simulink model "f_updated_vehicle_model"  (R2025b)
settings: Solver=ode23tb  StartTime=0.0  StopTime=20  MaxStep=0.001  RelTol=1e-3
model workspace (MAT data in the model file):
  init_r = 0
  init_vx = 0
  init_vy = 0
values from neighbouring files (symbols this model uses):
  Par =     [0_Load_data.mat]
  TireData =     [0_Load_data.mat]
undefined symbols (not defined in the file or in its folder): aero_par, Battery, Motor, SimInput_Steer, SimInput_TorqueFL, SimInput_TorqueFR, SimInput_TorqueRL, SimInput_TorqueRR, sus_par
libraries: simulink x3, BatteryEstimators x1
(part 2 of 2)

== matlab function f_updated_vehicle_model/roll and pitch angles/Phi_constants ==
  data: K_phi output; C_phi output; sus_par parameter; Par parameter
function [K_phi,C_phi] = fcn(sus_par,Par)

% Calculating Pitching stiffness
Kw_fl = sus_par.Ks_f.*(sus_par.Motion_ratio_f)^2; 
Kw_fr = sus_par.Ks_f.*(sus_par.Motion_ratio_f)^2;
Kw_rl = sus_par.Ks_r.*(sus_par.Motion_ratio_r)^2;
Kw_rr = sus_par.Ks_r.*(sus_par.Motion_ratio_r)^2;

K_phi = (Kw_fl + Kw_fr).*(Par.Tf/2)^2 + (Kw_rl + Kw_rr).*(Par.Tr/2)^2;

% Calculating Pitch Damping
Cw_fl = sus_par.C_damp_f.*(sus_par.Motion_ratio_f)^2;
Cw_fr = sus_par.C_damp_f.*(sus_par.Motion_ratio_f)^2;
Cw_rl = sus_par.C_damp_r.*(sus_par.Motion_ratio_r)^2;
Cw_rr = sus_par.C_damp_r.*(sus_par.Motion_ratio_r)^2;

C_phi = (Cw_fl + Cw_fr).*(Par.Tf/2)^2 + (Cw_rl + Cw_rr).*(Par.Tr/2)^2;

== matlab function f_updated_vehicle_model/Battery Pack/MATLAB Function ==
  data: Voc_pack input; v_bus output; R0_pack input; V_rc input; I_dc input
function v_bus = fcn(Voc_pack, R0_pack, V_rc, I_dc)
    % This function calculates the terminal voltage of the battery pack.
    % Voc_pack: Output from OCV LUT multiplied by Ns
    % R0_pack:  Output from R0 LUT multiplied by (Ns/Np)
    % V_rc:     Instantaneous voltage across the RC branch
    % I_dc:     Total DC current from the motor

    % 1. Calculate the instantaneous Ohmic drop (Ohm's Law)
    V_ohmic = I_dc * R0_pack;

    % 2. Calculate terminal voltage (Vt = Voc - V_ohmic - V_rc)
    v_bus = Voc_pack - V_ohmic - V_rc;

    % 3. Safety: Ensure voltage doesn't drop below a physical floor (e.g., 2.5V * Ns)
    % This prevents simulation crashes if the battery is fully depleted.
    v_bus = max(v_bus, 2.5 * 144); 
end

== matlab function f_updated_vehicle_model/Brakes/MATLAB Function ==
  data: brake_pedal input; T_brakes output; omega input; Brake parameter
function T_brakes = fcn(brake_pedal, omega, Brake)
    % BRAKE TORQUE CALCULATION
    % Converts normalized pedal/actuator position into physical torque
    % and ensures torque direction opposes wheel rotation.
    
    % 1. Calculate Magnitude of Torque based on Command (0-1)
    % We use the static max targets from the design sheet
    T_mag_Front = brake_pedal * Brake.MaxTorque_Wheel_F;
    T_mag_Rear  = brake_pedal * Brake.MaxTorque_Wheel_R;
    
    % Initialize output vector (FL, FR, RL, RR)
    T_brakes = zeros(1, 4);
    
    % 2. Apply Torque per Wheel with Directional Logic
    % Loop through all 4 wheels to apply logic individually
    % Indices: 1=FL, 2=FR, 3=RL, 4=RR
    
    for i = 1:4
        % Determine if this is a Front (1,2) or Rear (3,4) wheel
        if i <= 2
            T_req = T_mag_Front;
        else
            T_req = T_mag_Rear;
        end
        
        % Directional Check:
        % Torque must be negative if omega is positive, and vice versa.
        % -sign(omega) flips the torque direction.
        T_applied = T_req * -sign(omega(i));
        
        % Zero-Speed Cutoff:
        % If wheel is nearly stopped, clamp torque to zero to prevent 
        % the simulation from "driving" the car backwards.
        if abs(omega(i)) < Brake.ZeroSpeedThreshold
            T_applied = 0;
            
            % Advanced: Ideally, below threshold, T_brake should act as 
            % a viscous damper or Coulomb friction that exactly cancels 
            % remaining motion, but zeroing is sufficient for laptime sims.
        end
        
        T_brakes(i) = T_applied;
    end
end

== matlab function f_updated_vehicle_model/Motor/MATLAB Function ==
  data: rpm input; Torque_Nm output; throttle input; v_dc input
function Torque_Nm = fcn(rpm, throttle, v_dc)
    % 1. Constants
    p = 4;                      % Pole pairs 
    L = 0.393e-3;               % Inductance
    kt = 0.492;
    psi_m = kt/(1.5*p*sqrt(2));              % Flux linkage derived from kt
    I_lim = 61; % Peak phase current 
    V_max = v_dc / sqrt(3);     % Maximum available phase voltage
    
    % 2. Speed Conversion
    omega_m = rpm * (2*pi/60);
    omega_e = p * omega_m;
    
    % 3. MTPA / Field Weakening Logic
    if omega_e < 1e-3 % Handle standstill
        iq = I_lim* sqrt(2) * throttle;
        id = 0;
    else
        % Calculate required voltage for MTPA (id=0)
        V_req = omega_e * sqrt((L*I_lim)^2 + psi_m^2);
        
        if V_req <= V_max
            % Below base speed
            iq = I_lim;
            id = 0;
        else
            % Above base speed (Field Weakening)
            % Solving the quadratic for iq at the boundary of V_max and I_lim
            a = (omega_e * L)^2;
            b = 2 * omega_e^2 * L * psi_m;
            c = (omega_e * psi_m)^2 + (omega_e * L * I_lim)^2 - V_max^2;
            
            % Simple analytical approximation for constant power region
            iq = min(I_lim, V_max / (omega_e * L));
        end
    end
    
    % 4. Final Torque Calculation (with 29.1 Nm cap)
    Torque_Nm = min(29.1, 1.5 * p * psi_m * iq / sqrt(2)); 
end

== matlab function f_updated_vehicle_model/Normal Loads ==
  data: Fz_out output; phi input; theta input; Kw input; Vel input; Par parameter; Fs output size=4; Farb output; F_aero_total output; Zs output; aero_par parameter; sus_par parameter
function [Fz_out,Fs,Farb,F_aero_total,Zs] = fcn(phi,theta,Kw,Vel,Par,aero_par,sus_par)
    %#codegen
    % Inputs:
    %   ax_g, ay_g : Acceleration 
    %   m          : Mass [kg]
    %   Par        : Structure with field .g, .WB, .TW, .CG_h, .WD_R, .K_roll_F

    % 1. Constants
    g = Par.g;
    L = Par.WB;    % Wheelbase
    Tf = Par.Tf;   % Front track width
    Tr = Par.Tr;   % Rear Track width
    h = Par.CG_h;  % CG Height
    m = Par.m;
   
    % Front and rear Wheelbase
    Lf = L*0.51;  % Front wheel base
    Lr = L*0.49;  % Rear wheel base

    % Static load 
    F_static = m*g;  

    % Stiffness at each wheel:
    Kt = 90000;
    stiff_1 = Kw(1)*Kt/(Kw(1)+Kt);
    stiff_2 = Kw(2)*Kt/(Kw(2)+Kt);
    stiff_3 = Kw(3)*Kt/(Kw(3)+Kt);
    stiff_4 = Kw(4)*Kt/(Kw(4)+Kt);

    % F_aero = 0.5 * rho * Cl * A * v^2
    F_aero_total = -0.5 * aero_par.rho * aero_par.Cl * aero_par.Area * Vel^2;
    
    % Vertical deflection of each suspension(compression = -ve)
    zsfl = Lf*theta + (Tf/2)*phi - 0.5 * F_aero_total * (1 - aero_par.CP_rear)/stiff_1;
    zsfr = Lf*theta - (Tf/2)*phi - 0.5 * F_aero_total * (1 - aero_par.CP_rear)/stiff_2;
    zsrl = -Lr*theta + (Tr/2)*phi - 0.5 * F_aero_total*(aero_par.CP_rear)/stiff_3;
    zsrr = -Lr*theta - (Tr/2)*phi - 0.5 * F_aero_total*(aero_par.CP_rear)/stiff_4;

    Zs = [zsfl;zsfr;zsrl;zsrr];

    % Spring force at each wheel
    Fs_fl = stiff_1*zsfl;
    Fs_fr = stiff_2*zsfr;
    Fs_rl = stiff_3*zsrl;
    Fs_rr = stiff_4*zsrr;

    % Calculation of Anti roll bar forces at each wheel
    delta_zf = zsfl - zsfr;
    delta_zr = zsrl - zsrr;

    F_arb_fl = sus_par.K_arb_f*delta_zf/2;
    F_arb_fr = -sus_par.K_arb_f*delta_zf/2;
    F_arb_rl = sus_par.K_arb_r*delta_zr/2;
    F_arb_rr = -sus_par.K_arb_r*delta_zr/2;

    % Net normal force on each wheel
    F_static_per_wheel = F_static/4;

    Fz_FL = F_static_per_wheel - Fs_fl - F_arb_fl;
    Fz_FR = F_static_per_wheel - Fs_fr - F_arb_fr;
    Fz_RL = F_static_per_wheel - Fs_rl - F_arb_rl;
    Fz_RR = F_static_per_wheel - Fs_rr - F_arb_rr;
   
    % Safety Clamp (Wheelie prevention)
    Min_Load = 10; 

    Fz_FL = max(Fz_FL, Min_Load);
    Fz_FR = max(Fz_FR, Min_Load);
    Fz_RL = max(Fz_RL, Min_Load);
    Fz_RR = max(Fz_RR, Min_Load);

    Fz_out = [Fz_FL; Fz_FR; Fz_RL; Fz_RR];
    
    Fs = [Fs_fl;Fs_fr;Fs_rl;Fs_rr];
    Farb = [F_arb_fl;F_arb_fr;F_arb_rl;F_arb_rr];

% Distribute Aero (Usually based on Center of Pressure, CP)
   % 
   % aero_Fz_FL = Fz_FL + ;
   % aero_Fz_FR = Fz_FR + ;
   % aero_Fz_RL = Fz_RL + ;
   % aero_Fz_RR = Fz_RR + ;

   % Fz_new = [aero_Fz_FL;aero_Fz_FR;aero_Fz_RL;aero_Fz_RR];
   
   
end

== matlab function f_updated_vehicle_model/Motor/MATLAB Function1 ==
  data: rpm_feedback input; Torque_Nm output; throttle input; v_dc_bus input
function Torque_Nm = fcn(rpm_feedback, throttle, v_dc_bus)
    % --- 1. Define Motor Constants from Datasheet ---
    p = 4;                          % Number of pole pairs 
    L = 0.393e-3;                   % Phase inductance in Henries 
    kt = 0.492;                     % Torque constant in Nm/Arms 
    psi_m = kt / (1.5 * p * sqrt(2)); % Calculate magnet flux linkage (~0.058 Wb)
    I_max_rms = 61;                 % Maximum peak current in Arms 
    n_max = 20000;                  % Maximum mechanical RPM limit 
    T_peak_limit = 29.1;            % Absolute peak torque cap in Nm 

    % --- 2. Enforce Hard Mechanical RPM Limit ---
    if abs(rpm_feedback) >= n_max   % Check if current speed exceeds mechanical redline
        Torque_Nm = 0;              % Kill all torque production at the limit
        return;                     % Exit function immediately
    end

    % --- 3. Convert Inputs to Electrical Units ---
    omega_m = rpm_feedback * (2*pi/60);      % Convert mechanical RPM to rad/s
    omega_e = omega_m * p;                   % Convert mechanical speed to electrical frequency
    V_max_phase = v_dc_bus / sqrt(3);        % Calculate max phase voltage (fundamental limit)
    I_cmd_peak = I_max_rms * sqrt(2) * throttle; % Scaled peak current command based on throttle

    % --- 4. Determine Operating Region (MTPA vs. Field Weakening) ---
    % Calculate the voltage required for MTPA (where id = 0)
    % Equation: V = omega_e * sqrt( (L*iq)^2 + (psi_m)^2 )
    V_required_mtpa = abs(omega_e) * sqrt((L * I_cmd_peak)^2 + psi_m^2);

    if V_required_mtpa <= V_max_phase        % If enough voltage is available for requested torque
        % REGION 1: Below Base Speed (Maximum Torque Per Ampere)
        id = 0;                              % No d-axis current needed (standard operation)
        iq = I_cmd_peak;                     % All available current used for torque production
    else
        % REGION 2: Above Base Speed (Field Weakening)
        % We must inject negative d-axis current (id) to oppose psi_m and stay within V_max
        % Intersection of Current Circle (id^2 + iq^2 = I^2) and Voltage Ellipse
        
        % Solving the voltage ellipse for id:
        % (V_max/omega_e)^2 = (L*iq)^2 + (L*id + psi_m)^2
        % This simplifies to a quadratic equation for id
        a_quad = L^2;                        % Quadratic coefficient 'a'
        b_quad = 2 * L * psi_m;              % Quadratic coefficient 'b'
        c_quad = psi_m^2 + (L * I_cmd_peak)^2 - (V_max_phase / omega_e)^2; % Coefficient 'c'
        
        % Calculate the required negative d-axis current using the quadratic formula
        id = (-b_quad + sqrt(b_quad^2 - 4 * a_quad * c_quad)) / (2 * a_quad);
        
        % Enforce physical bounds on current components
        id = max(min(id, 0), -I_cmd_peak);   % Clamp id between -I_max and 0
        iq = sqrt(max(0, I_cmd_peak^2 - id^2)); % Solve for remaining q-axis current
    end

    % --- 5. Calculate Final Torque Output ---
    % Standard PMSM Torque Equation: Te = 1.5 * p * psi_m * iq
    T_generated = 1.5 * p * psi_m * iq;      % Calculate the raw electromagnetic torque
    
    % Final output is capped by the mechanical peak torque of the motor
    Torque_Nm = min(T_generated, T_peak_limit); % Saturate at 29.1 Nm 
end

== matlab function f_updated_vehicle_model/Motor/Motor with Field Weakening ==
  data: rpm_feedback input; Torque_Nm output; throttle input; v_dc_bus input; Motor parameter; I_dc output
function [Torque_Nm, I_dc] = fcn(rpm_feedback, throttle, v_dc_bus, Motor)
    % HIGH-FIDELITY PMSM MOTOR MODEL
    % Inputs:
    %   rpm_feedback : Instantaneous wheel speed * gear ratio [rpm]
    %   throttle     : Driver input signal [0 to 1]
    %   v_dc_bus     : Instantaneous voltage from battery pack [V]
    %   Motor        : Struct containing constants (kt, L, p, n_max, etc.)
    
    % --- 1. Enforce Mechanical Redline ---
    % n_max is 20,000 rpm per datasheet.
    if abs(rpm_feedback) >= Motor.n_max
        Torque_Nm = 0;
        I_dc = 0;
        return;
    end

    % --- 2. Electrical Conversions ---
    omega_m = rpm_feedback * (2*pi/60);          % Mechanical rad/s
    omega_e = abs(omega_m * Motor.p);            % Electrical frequency 
    V_max_phase = v_dc_bus / sqrt(3);            % Max phase voltage (fundamental limit)
    I_cmd_peak = Motor.I_max_rms * sqrt(2) * throttle; % Commanded peak current 

    % --- 3. Region Selection: MTPA vs Field Weakening ---
    % Calculate voltage required for id=0 operation (Maximum Torque Per Ampere)
    % psi_m is the flux linkage derived from kt (~0.492 Nm/A).
    V_req_mtpa = omega_e * sqrt((Motor.L * I_cmd_peak)^2 + Motor.psi_m^2);

    if V_req_mtpa <= V_max_phase
        % REGION 1: Below Base Speed
        id = 0;
        iq = I_cmd_peak;
    else
        % REGION 2: Above Base Speed (Field Weakening)
        % Intersecting the Current Circle (id^2 + iq^2 = Imax^2) with the Voltage Ellipse.
        % Solving the quadratic for d-axis current (id).
        a = Motor.L^2;
        b = 2 * Motor.L * Motor.psi_m;
        c = Motor.psi_m^2 + (Motor.L * I_cmd_peak)^2 - (V_max_phase / max(omega_e(3), 0.1))^2;
        
        % Solve for negative id to oppose magnet flux
        id = (-b + sqrt(b^2 - 4 * a * c)) / (2 * a);
        
        % Ensure id is within physical bounds and calculate remaining iq
        id = max(min(id, 0), -I_cmd_peak); 
        iq = sqrt(max(0, I_cmd_peak^2 - id^2));
    end

    % --- 4. Torque Calculation ---
    % Te = 1.5 * p * psi_m * iq
    T_generated = 1.5 * Motor.p * Motor.psi_m * iq;
    
    % Cap at peak mechanical torque (29.1 Nm)[cite: 8, 136].
    Torque_Nm = min(T_generated, Motor.T_peak_limit);

    % --- 5. DC Current Calculation (The Battery Interaction) ---
    % Mechanical Output Power
    P_mech = abs(Torque_Nm * omega_m(3));
    
    % Copper Losses (3 * R_phase * I_rms^2) 
    % R_phase = 0.126 Ohm per datasheet.
    P_copper = 3 * 0.126 * (I_cmd_peak / sqrt(2))^2;
    
    % Total electrical power requested from the battery
    P_elec_total = P_mech + P_copper;
    
    % Calculate DC current draw (I = P/V)
    if v_dc_bus > 10
        I_dc = P_elec_total / v_dc_bus;
    else
        I_dc = 0;
    end
end

== matlab function f_updated_vehicle_model/Torque Distribution/MATLAB Function ==
  data: T_wheel input; T_FL output; T_brake_vec input; T_FR output; T_RL output; T_RR output
function [T_FL, T_FR, T_RL, T_RR] = torque_combiner(T_wheel, T_brake_vec)
    % T_brake_vec is a 4x1 input: [FL; FR; RL; RR]
    
    % Front Wheels: Brake only
    T_FL = -T_brake_vec(1);
    T_FR = -T_brake_vec(2);
    
    % Rear Wheels: (Motor / 2) - Brake
    % Assuming 50/50 torque split from an open diff
    T_RL = (T_wheel) - T_brake_vec(3);
    T_RR = (T_wheel) - T_brake_vec(4);
end

== matlab function f_updated_vehicle_model/Simplified Tire Model ==
  data: Fz input; Fx output size=4; slip_ratios input; slip_angles input; camber_angles input; Fy output size=4; Mz output size=4; Mu_x output size=4; Mu_y output size=4; TireData parameter; Par parameter; sus_par parameter
function [Fx, Fy, Mz, Mu_x, Mu_y] = fcn(Fz, slip_ratios, slip_angles, camber_angles, TireData,Par,sus_par)
%#codegen
% =========================================================================
%  VECTORIZED MAGIC FORMULA 5.2 (4-WHEEL)
%  Computes tire physics for all 4 corners simultaneously using element-wise math.
%
%  INPUTS (All 4x1 Vectors):
%    Fz    : Vertical Loads [N] -> [FL; FR; RL; RR]
%    Kappa : Slip Ratios [-]
%    Alpha : Slip Angles [rad]
%    Gamma : Camber Angles [rad]
%    TireData : Parameter Struct (Must be loaded in Base Workspace)
%
%  OUTPUTS (All 4x1 Vectors):
%    Fx    : Longitudinal Force [N]
%    Fy    : Lateral Force [N]
%    Mz    : Self-Aligning Torque [Nm]
%    Mu_x  : Long. Friction Coeff [-]
%    Mu_y  : Lat. Friction Coeff [-]
% =========================================================================

    % 1. EXTRACT PARAMETERS (Scalars)
    p = TireData;
    s = TireData.Scales;
    Fz0 = Par.Fz0;
    Rw  = Par.R0;
    
    % 2. INPUT SAFETY & NORMALIZATION
    % Clamp negative loads to 0 (Tires can't pull ground)
    Fz_safe = max(Fz, 0); 
    
    % Avoid division by zero for Mu calculations later
    Fz_denom = max(Fz_safe, 1.0); 

    % Normalized Load (dfz) - Vectorized
    dfz = (Fz_safe - Fz0) ./ Fz0;

    % ---------------------------------------------------------------------
    % A. LONGITUDINAL FORCE (Fx) - VECTORIZED
    % ---------------------------------------------------------------------
    Cx = p.PCX1 * s.LCX;
    
    % Friction Coeff Mu_x
    mu_x_base = (p.PDX1 + p.PDX2 .* dfz) .* (1 - p.PDX3 .* camber_angles.^2) .* s.LMUX;
    Dx = mu_x_base .* Fz_safe;
    
    % Stiffness Kx
    Kx = Fz_safe .* (p.PKX1 + p.PKX2 .* dfz) .* exp(p.PKX3 .* dfz) .* s.LKX;
    
    % Stiffness Factor Bx
    Bx = Kx ./ (Cx .* Dx + 1e-6); 
    
    % Shifts (Horizontal & Vertical)
    Shx = (p.PHX1 + p.PHX2 .* dfz) .* s.LHX;
    Svx = Fz_safe .* (p.PVX1 + p.PVX2 .* dfz) .* s.LVX;
    
    % Composite Slip
    k_s = slip_ratios + Shx;
    
    % Curvature Ex (Sign Dependent)
    Ex = (p.PEX1 + p.PEX2 .* dfz + p.PEX3 .* dfz.^2) .* (1 - p.PEX4 .* sign(k_s)) .* s.LEX;
    Ex(Ex > 1) = 1; % Clamp
    
    % Calculation
    Bx_k = Bx .* k_s;
    Fx = Dx .* sin(Cx .* atan(Bx_k - Ex .* (Bx_k - atan(Bx_k)))) + Svx;

    % ---------------------------------------------------------------------
    % B. LATERAL FORCE (Fy) - VECTORIZED
    % ---------------------------------------------------------------------
    Cy = p.PCY1 * s.LCY;
    
    % Friction Coeff Mu_y
    mu_y_base = (p.PDY1 + p.PDY2 .* dfz) .* (1 - p.PDY3 .* camber_angles.^2) .* s.LMUY;
    Dy = mu_y_base .* Fz_safe;
    
    % Cornering Stiffness Ky (Trig Form)
    Ky = p.PKY1 .* Fz0 .* sin(2 .* atan(Fz_safe ./ (p.PKY2 .* Fz0))) .* (1 - p.PKY3 .* abs(camber_angles)) .* s.LKY;
    
    % Poly fallback check (if PKY2 implies poly form)
    if (Ky(1) < 1)
        Ky = Fz_safe .* (p.PKY1 + p.PKY2 .* dfz) .* s.LKY;
    end
    
    By = Ky ./ (Cy .* Dy + 1e-6);
    
    % Shifts
    Shy = (p.PHY1 + p.PHY2 .* dfz) .* s.LHY;
    Svy = Fz_safe .* (p.PVY1 + p.PVY2 .* dfz) .* s.LVY;
    
    a_s = slip_angles + 0*Shy;
    
    % Curvature Ey (Sign Dependent)
    Ey = (p.PEY1 + p.PEY2 .* dfz) .* (1 - (p.PEY3 + p.PEY4 .* camber_angles) .* sign(a_s)) .* s.LEY;
    Ey(Ey > 1) = 1;
    
    % Calculation
    By_a = By .* a_s;
    Fy = -(Dy .* sin(Cy .* atan(By_a - Ey .* (By_a - atan(By_a)))) + 0*Svy);

    % ---------------------------------------------------------------------
    % C. SELF-ALIGNING TORQUE (Mz) - VECTORIZED
    % ---------------------------------------------------------------------
    % Peak Trail Dt
    Dt = (p.QDZ1 + p.QDZ2 .* dfz) .* (1 - p.QDZ3 .* abs(camber_angles)) .* Rw .* s.LTR;
    
    % Trail Slope Bt
    Bt = (p.QBZ1 + p.QBZ2 .* dfz + p.QBZ3 .* dfz.^2) .* (1 + p.QBZ4 .* abs(camber_angles)) .* (s.LKY / s.LMUY);
    
    Ct = p.QCZ1; % Scalar
    Et = (p.QEZ1 + p.QEZ2 .* dfz + p.QEZ3 .* dfz.^2);
    
    % Trail 't' Calculation(Pneumatic trail)
    Bt_a = Bt .* a_s;
    alpha_t = Bt_a - Et .* (Bt_a - atan(Bt_a));
    t = Dt .* cos(Ct .* atan(alpha_t)) .* cos(a_s);

    % Trail 'tm' Calculation(mechanical trail)
    tm = Rw.*tan(sus_par.Caster_static);

    % Residual Mzr
    Dr = Fz_safe .* Rw .* (p.QDZ6 + p.QDZ7 .* dfz) .* s.LRES;
    Br = 10;
    Mzr = Dr .* cos(atan(Br .* a_s));
    
    % Final Mz (Standard Restoring: Negative Slope)
    % Note: If you want positive slope (sharp tune from before), multiply term by -1.
    Mz = -(t+tm).*Fy + Mzr;

    % ---------------------------------------------------------------------
    % D. OUTPUTS (Zero out lifted wheels)
    % ---------------------------------------------------------------------
    % Friction Coeffs
    Mu_x = Fx ./ Fz_denom;
    Mu_y = Fy ./ Fz_denom;

    % Clean up lifted wheels (Fz <= 0)
    % lifted_idx = Fz <= 0;
    % Fx(lifted_idx) = 0;
    % Fy(lifted_idx) = 0;
    % Mz(lifted_idx) = 0;
    % Mu_x(lifted_idx) = 0;
    % Mu_y(lifted_idx) = 0;

end

== matlab function f_updated_vehicle_model/slip ratios ==
  data: Vx input; Vy input; slip_ratios output; yawrate input; Omega input; Steer_FL input; Steer_FR input; Par parameter
function slip_ratios = fcn(Vx,Vy, yawrate, Omega,Steer_FL,Steer_FR, Par)
%#codegen


    % 1. Constants
    Tf = Par.Tf;
    Tr = Par.Tr;
    Rw = Par.R0;
    
    a = Par.Lf;
    b = Par.Lr;
    r = yawrate;
    % 2 Yaw Rate Correction (Kinematics)
    
    Vx_FL = Vx - yawrate * (Tf/2);  % Front Left
    Vx_FR = Vx + yawrate * (Tf/2);  % Fron Right
    Vx_RL = Vx - yawrate * (Tr/2);  % Rear Left
    Vx_RR = Vx + yawrate * (Tr/2);  % Rear Right
    
    Vx_vec = [Vx_FL; Vx_FR; Vx_RL; Vx_RR];
    
    Vy_FL = Vy + r * a;
    Vy_FR = Vy+ r * a;
    Vy_RL = Vy- r * b;
    Vy_RR = Vy- r * b;

    Vy_vec = [Vy_FL; Vy_FR; Vy_RL; Vy_RR];
    Delta = [Steer_FL;Steer_FR;0;0];
    % 3. Slip Angle Correction (Projection)
 
    V_road_plane = Vx_vec .* cos(Delta) + Vy_vec .* sin(Delta);

    % 4. Calculate Wheel Linear Speed
    V_wheel = Omega .* Rw;

    % 5. Calculate Slip Ratio
    V_safe_threshold = 0.1; 
    V_ref = max(abs(V_road_plane), V_safe_threshold);
    
    slip_ratios_raw = (V_wheel - V_road_plane) ./ V_ref;
    slip_ratios = min(max(slip_ratios_raw,-1),1);
end

== matlab function f_updated_vehicle_model/Slip Angles ==
  data: Vx input; slip_angles output; Vy input; yawrate input; Steer_FL input; Steer_FR input; Par parameter
function slip_angles = fcn(Vx, Vy, yawrate, Steer_FL, Steer_FR, Par)
%#codegen

    % 1. Geometry Setup
    T = Par.Tf;
    
    % Distance from CG to Axles
    a = Par.Lf;     
    b = Par.Lr;             
    half_T = T / 2;

    % 2. Calculate Velocity Components at Each Corner
    % Kinematic transformation from CG to Hubs
    % Front Left (1)
        Vx_FL = Vx - yawrate * half_T;
        Vy_FL = Vy + yawrate * a;
    
    % Front Right (2)
        Vx_FR = Vx + yawrate * half_T;
        Vy_FR = Vy + yawrate * a;
    
    % Rear Left (3)
        Vx_RL = Vx - yawrate * half_T;
        Vy_RL = Vy - yawrate * b;
    
    % Rear Right (4)
        Vx_RR = Vx + yawrate * half_T;
        Vy_RR = Vy - yawrate * b;

    % 3. Calculate Velocity Angles (Theta_V)

        Theta_FL = atan2(Vy_FL, max(Vx_FL,0.1)); 
        Theta_FR = atan2(Vy_FR, max(Vx_FR,0.1));
        Theta_RL = atan2(Vy_RL, max(Vx_RL,0.1));
        Theta_RR = atan2(Vy_RR, max(Vx_RR,0.1));
    
    % 4. Construct Steering Vector (Delta)
    % Rears are assumed fixed (0 steering)
        Delta = [Steer_FL; Steer_FR; 0; 0];
    
    % Vector of Velocity Angles
        Theta_V = [Theta_FL; Theta_FR; Theta_RL; Theta_RR];

    % 5. Final Calculation
    % Alpha = Delta - Theta_V
        slip_angles = Delta - Theta_V ;
end

== matlab function f_updated_vehicle_model/Wheel to Vehicle Coordinates ==
  data: Fx_w input; Fx_b output; Fy_w input; Steer_FL input; Steer_FR input; Fy_b output; B_Fx output; B_Fy output
function [Fx_b, Fy_b, B_Fx, B_Fy] = fcn(Fx_w, Fy_w, Steer_FL, Steer_FR)
%#codegen
% FORCE & MOMENT RESOLVER
    % 1. Construct Steering Vector [FL; FR; RL; RR]
    % Rear steering is assumed to be 0
    Delta = [Steer_FL; Steer_FR; 0; 0];
    
    % 2. Pre-calculate Trig functions (Vectorized)
    c_d = cos(Delta);
    s_d = sin(Delta);
    
    % Longitudinal Body Force:

    Fx_b = Fx_w .* c_d - Fy_w .* s_d;
    
    % Lateral Body Force:
    % Fy_body = Fx_wheel * sin(delta) + Fy_wheel * cos(delta)
    Fy_b = Fx_w .* s_d + Fy_w .* c_d;
    
    % 4. Summation: Total Forces acting on CG
    B_Fx = sum(Fx_b);
    B_Fy = sum(Fy_b);
    
end

== matlab function f_updated_vehicle_model/Steering Kinematics/Steering Kinematics ==
  data: Steer_Input input; Ackermann_Pct input; Steer_FL output; Steer_FR output; Par parameter
function [Steer_FL, Steer_FR] = fcn(Steer_Input, Ackermann_Pct, Par)
%#codegen

    % 1. Constants
    L = Par.WB;      % Wheelbase
    half_T = Par.Tf / 2; % Half Track Width

    % 2. Safety Clamp (Prevent tan(90) singularity)
    delta = min(max(Steer_Input, -1.5), 1.5); 
    
    % 3. Calculate "Pure Ackermann" Angles
    % Ideally, inner wheel turns sharper than outer wheel.
    tan_d = tan(delta);
    
    % FL (Left): Denom depends on sign of turn.
    % If turning Left (+), Denom shrinks (Sharper).
    FL_Ack = atan( (L * tan_d) / (L - half_T * tan_d) );
    
    % FR (Right): 
    % If turning Left (+), Denom grows (Shallower).
    FR_Ack = atan( (L * tan_d) / (L + half_T * tan_d) );
    
    % 4. Calculate "Parallel" Angles
    % Both wheels exactly match the center input
    FL_Par = delta;
    FR_Par = delta;
    
    % 5. Linear Blend based on Percentage
    % Formula: Final = Parallel + (Ackermann - Parallel) * Percent
    Steer_FL = FL_Par + (FL_Ack - FL_Par) * Ackermann_Pct;
    Steer_FR = FR_Par + (FR_Ack - FR_Par) * Ackermann_Pct;

end
